simulink library "sm_vehicle_utilities_lib"  (R2024b)
settings: Solver=VariableStepAuto  StartTime=0.0  StopTime=10.0  RelTol=1e-3
undefined symbols (not defined in the file): Camera, Init, LorR, mu_surface, p1, p2, Scene_Data, SceneData, tire_data_205_60R19, vehdata, X, Y, Z
libraries: sm_lib x90, nesl_utility x49, $bdroot x33, fl_lib x10, simulink x8
(part 2 of 3)

== system sm_vehicle_utilities_lib/Mesh ==
  Solid : sm_lib/Body Elements/Extruded Solid  ExtrusionType=General  PolygonNumSides=3  PolygonOuterRadius=1  PolygonOuterRadiusUnits=m  ExportEntireGeometry=off  ExtrusionCrossSection=mesh_xsec  ExtrusionCrossSectionUnits=m  ExportConvexHullGeometry=off  ExtrusionLength=mesh_thickness  ExtrusionLengthUnits=m  InertiaType=CalculateFromGeometry  BasedOnType=Density  Density=mesh_rho  DensityUnits=kg/(m^3)  Mass=1  MassUnits=kg  CenterOfMass=[0 0 0]  CenterOfMassUnits=m  MomentsOfInertia=[1 1 1]  MomentsOfInertiaUnits=kg*m^2  ProductsOfInertia=[0 0 0]  ProductsOfInertiaUnits=kg*m^2  GraphicType=FromGeometry  MarkerShape=Sphere  MarkerSize=10  GraphicVisPropType=SimpleVisualProperties  GraphicDiffuseColor=mesh_color  GraphicOpacity=mesh_opc  GraphicSpecularColor=[0.5 0.5 0.5 1.0]  GraphicAmbientColor=[0.15 0.15 0.15 1.0]  GraphicEmissiveColor=[0.0 0.0 0.0 1.0]  GraphicShininess=75  DoExposeReferenceFrame=on  SerializedFrames=<Frames><Frame><Id>Frame1</Id><Value><Name>F</Name><Origin><Source>GeometricFeature</Source><FeatureName>top surface</FeatureName></Origin><PrimaryAxis><DefinedDirection>+Z</DefinedDirection><Source>ReferenceFrame</Source><SourceDirection>+Z</SourceDirection><FeatureName></FeatureName></PrimaryAxis><SecondaryAxis><DefinedDirection>+X</DefinedDirection><Source>ReferenceFrame</Source><SourceDirection>+X</SourceDirection><FeatureName></FeatureName></SecondaryAxis></Value></Frame><Frame><Id>Frame2</Id><Value><Name>B</Name><Origin><Source>GeometricFeature</Source><FeatureName>bottom surface</FeatureName></Origin><PrimaryAxis><DefinedDirection>+Z</DefinedDirection><Source>ReferenceFrame</Source><SourceDirection>+Z</SourceDirection><FeatureName></FeatureName></PrimaryAxis><SecondaryAxis><DefinedDirection>+X</DefinedDirection><Source>ReferenceFrame</Source><SourceDirection>+X</SourceDirection><FeatureName></FeatureName></SecondaryAxis></Value></Frame></Frames>
  F : PMIOPort  Side=Right
  R : PMIOPort  Port=2  Side=Left
  B : PMIOPort  Port=3  Side=Right
  connections:
  B/RConn1 -- Solid/LConn2
  F/RConn1 -- Solid/LConn1
  Solid/RConn1 -- R/RConn1

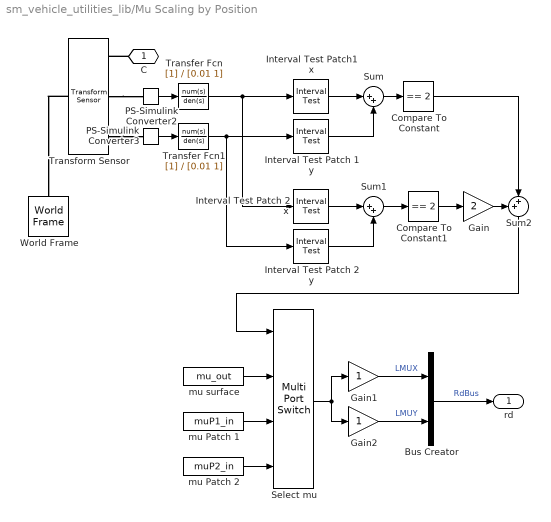
== system sm_vehicle_utilities_lib/Mu Scaling by Position ==
  Bus Creator : BusCreator  Inputs=2
  Compare To Constant : simulink/Logic and Bit Operations/Compare To Constant  relop===  const=2  OutDataTypeStr=boolean  ZeroCross=off
  Compare To Constant1 : simulink/Logic and Bit Operations/Compare To Constant  relop===  const=2  OutDataTypeStr=boolean  ZeroCross=off
  Gain : Gain  Gain=2
  Gain1 : Gain
  Gain2 : Gain
  Interval Test Patch 1 y : simulink/Logic and Bit Operations/Interval Test  IntervalClosedRight=on  uplimit=intvY_P1_end  IntervalClosedLeft=on  lowlimit=intvY_P1_start  OutDataTypeStr=uint8
  Interval Test Patch 2 x : simulink/Logic and Bit Operations/Interval Test  IntervalClosedRight=on  uplimit=intvX_P2_end  IntervalClosedLeft=on  lowlimit=intvX_P2_start  OutDataTypeStr=uint8
  Interval Test Patch 2 y : simulink/Logic and Bit Operations/Interval Test  IntervalClosedRight=on  uplimit=intvY_P2_end  IntervalClosedLeft=on  lowlimit=intvY_P2_start  OutDataTypeStr=uint8
  Interval Test Patch1 x : simulink/Logic and Bit Operations/Interval Test  IntervalClosedRight=on  uplimit=intvX_P1_end  IntervalClosedLeft=on  lowlimit=intvX_P1_start  OutDataTypeStr=uint8
  PS-Simulink Converter2 : nesl_utility/PS-Simulink Converter  PhysicalDomain=network_engine_domain  SubClassName=ps_output  LeftPortType=input  RightPortType=output  PseudoPeriodic=off  Frequencies=[]  VectorFormat=inherit  Unit=inherit  AffineConversion=off
  PS-Simulink Converter3 : nesl_utility/PS-Simulink Converter  PhysicalDomain=network_engine_domain  SubClassName=ps_output  LeftPortType=input  RightPortType=output  PseudoPeriodic=off  Frequencies=[]  VectorFormat=inherit  Unit=inherit  AffineConversion=off
  Select mu : MultiPortSwitch  DataPortOrder=Zero-based contiguous  zeroidx=on  SaturateOnIntegerOverflow=off  InputSameDT=off
  Sum : Sum  Inputs=|++
  Sum1 : Sum  Inputs=|++
  Sum2 : Sum  Inputs=++|
  Transfer Fcn : TransferFcn  Denominator=[0.01 1]
  Transfer Fcn1 : TransferFcn  Denominator=[0.01 1]
  Transform Sensor : sm_lib/Frames and Transforms/Transform Sensor  MeasurementFrame=World  RotationSequence=XYX  SenseAngle=off  SenseAxis=off  SenseQ=off  SenseR=off  SenseRotationSequence=off  SenseOmegaX=off  SenseOmegaY=off  SenseOmegaZ=off  SenseOmega=off  SenseQDot=off  SenseRDot=off  SenseRotationSequenceDot=off  SenseAlphaX=off  SenseAlphaY=off  SenseAlphaZ=off  SenseAlpha=off  SenseQDDot=off  SenseRDDot=off  SenseX=on  SenseY=on  SenseZ=off  SenseXYZ=off  SenseRad=off  SenseAzim=off  SenseDist=off  SenseInc=off  SenseXDot=off  SenseYDot=off  SenseZDot=off  SenseXYZDot=off  SenseRadDot=off  SenseAzimDot=off  SenseDistDot=off  SenseIncDot=off  SenseXDDot=off  SenseYDDot=off  SenseZDDot=off  SenseXYZDDot=off  SenseRadDDot=off  SenseAzimDDot=off  SenseDistDDot=off  SenseIncDDot=off
  World Frame : sm_lib/Frames and Transforms/World Frame
  mu Patch 1 : Constant  Value=muP1_in
  mu Patch 2 : Constant  Value=muP2_in
  mu surface : Constant  Value=mu_out
  C : PMIOPort  Side=Right
  rd : Outport  VectorParamsAs1DForOutWhenUnconnected=off
  wires:
  Interval Test Patch 2 y/1 -> Sum1/2
  Transfer Fcn1/1 -> Interval Test Patch 2 y/1, Interval Test Patch 1 y/1
  Sum1/1 -> Compare To Constant1/1
  Transfer Fcn/1 -> Interval Test Patch 2 x/1, Interval Test Patch1 x/1
  Interval Test Patch 2 x/1 -> Sum1/1
  Interval Test Patch1 x/1 -> Sum/1
  Interval Test Patch 1 y/1 -> Sum/2
  Sum/1 -> Compare To Constant/1
  Compare To Constant1/1 -> Gain/1
  mu surface/1 -> Select mu/2
  mu Patch 1/1 -> Select mu/3
  mu Patch 2/1 -> Select mu/4
  Sum2/1 -> Select mu/1
  Select mu/1 -> Gain2/1, Gain1/1
  Gain1/1 -> Bus Creator/1  "LMUX"
  Gain2/1 -> Bus Creator/2  "LMUY"
  Bus Creator/1 -> rd/1  "RdBus"
  Compare To Constant/1 -> Sum2/2
  Gain/1 -> Sum2/1
  PS-Simulink Converter2/1 -> Transfer Fcn/1
  PS-Simulink Converter3/1 -> Transfer Fcn1/1
  connections:
  C/RConn1 -- Transform Sensor/RConn1
  Transform Sensor/LConn1 -- World Frame/RConn1
  Transform Sensor/RConn2 -- PS-Simulink Converter2/LConn1
  Transform Sensor/RConn3 -- PS-Simulink Converter3/LConn1

== system sm_vehicle_utilities_lib/Pad Rotor ==
  note: Separate hard stop blocks are used so that we can measure only the pressure the piston applies to the rotor and so that we can have different stiffness values for piston-rotor and piston-caliper housing.
  note: Newtons
  note: Pascal
  Force Sensor : fl_lib/Mechanical/Mechanical Sensors/Ideal Force Sensor
  Hard Stop Caliper : fl_lib/Mechanical/Translational Elements/Translational Hard Stop  upper_bnd=0.1 m  lower_bnd=0 m  model=1  stiff_up=1e6 N/m  stiff_low=1e6 N/m  D_up=150 N/(m/s)  D_low=150 N/(m/s)  transition=0.1 mm  coeff_rest=0.7  v_tol=0.001 m/s  f_tol=0.001 N  v_specify=off  v_priority=None  v=0 m/s  v_nominal_specify=off  v_nominal_value=1  v_nominal_unit=m/s  f_specify=off  f_priority=None  f=0 N  f_nominal_specify=off  f_nominal_value=1  f_nominal_unit=N  x_specify=off  x_priority=High  x=0 m  x_nominal_specify=off  x_nominal_value=1  x_nominal_unit=m  M_specify=off  M_priority=None  M=0
  Hard Stop Rotor : fl_lib/Mechanical/Translational Elements/Translational Hard Stop  upper_bnd=0.45*1e-3 m  lower_bnd=-0.1 m  model=1  stiff_up=1e9*1e-3 N/m  stiff_low=1e9*1e-3 N/m  D_up=1e6*1e-3 N/(m/s)  D_low=1e6*1e-3 N/(m/s)  transition=0.045*1e-3 m  coeff_rest=0.7  v_tol=0.001 m/s  f_tol=0.001 N  v_specify=off  v_priority=None  v=0 m/s  v_nominal_specify=off  v_nominal_value=1  v_nominal_unit=m/s  f_specify=off  f_priority=None  f=0 N  f_nominal_specify=off  f_nominal_value=1  f_nominal_unit=N  x_specify=off  x_priority=High  x=0 m  x_nominal_specify=off  x_nominal_value=1  x_nominal_unit=m  M_specify=off  M_priority=None  M=0
  MTRef : fl_lib/Mechanical/Translational Elements/Mechanical Translational Reference
  MTRef1 : fl_lib/Mechanical/Translational Elements/Mechanical Translational Reference
  Mass : fl_lib/Mechanical/Translational Elements/Mass  mass=0.3 kg  num_ports=foundation.enum.numPorts2.one  v_specify=off  v_priority=High  v=0 m/s  v_nominal_specify=off  v_nominal_value=1  v_nominal_unit=m/s  f_specify=off  f_priority=None  f=0 N  f_nominal_specify=off  f_nominal_value=1  f_nominal_unit=N
  PS Calc Pressure Rotor : fl_lib/Physical Signals/Functions/PS Divide
  PS Cyl A : Subsystem
  pPad : PMIOPort  Side=Left
  Piston : PMIOPort  Port=2  Side=Right
  connections:
  PS Calc Pressure Rotor/RConn1 -- pPad/RConn1
  PS Calc Pressure Rotor/LConn2 -- PS Cyl A/RConn1
  PS Calc Pressure Rotor/LConn1 -- Force Sensor/RConn2
  Hard Stop Rotor/RConn1 -- Force Sensor/LConn1
  Force Sensor/RConn1 -- MTRef/LConn1
  Piston/RConn1 -- Hard Stop Rotor/LConn1 -- Hard Stop Caliper/LConn1 -- Mass/LConn1
  MTRef1/LConn1 -- Hard Stop Caliper/RConn1

== system sm_vehicle_utilities_lib/Plateau ==
  PS-Simulink Converter2 : nesl_utility/PS-Simulink Converter  PhysicalDomain=network_engine_domain  SubClassName=ps_output  LeftPortType=input  RightPortType=output  PseudoPeriodic=off  Frequencies=[]  VectorFormat=inherit  Unit=inherit  AffineConversion=off
  PS-Simulink Converter3 : nesl_utility/PS-Simulink Converter  PhysicalDomain=network_engine_domain  SubClassName=ps_output  LeftPortType=input  RightPortType=output  PseudoPeriodic=off  Frequencies=[]  VectorFormat=inherit  Unit=inherit  AffineConversion=off
  Road : Subsystem
  Transfer Fcn : TransferFcn  Denominator=[0.01 1]
  Transfer Fcn1 : TransferFcn  Denominator=[0.01 1]
  Transform Sensor : sm_lib/Frames and Transforms/Transform Sensor  MeasurementFrame=World  RotationSequence=XYX  SenseAngle=off  SenseAxis=off  SenseQ=off  SenseR=off  SenseRotationSequence=off  SenseOmegaX=off  SenseOmegaY=off  SenseOmegaZ=off  SenseOmega=off  SenseQDot=off  SenseRDot=off  SenseRotationSequenceDot=off  SenseAlphaX=off  SenseAlphaY=off  SenseAlphaZ=off  SenseAlpha=off  SenseQDDot=off  SenseRDDot=off  SenseX=on  SenseY=on  SenseZ=off  SenseXYZ=off  SenseRad=off  SenseAzim=off  SenseDist=off  SenseInc=off  SenseXDot=off  SenseYDot=off  SenseZDot=off  SenseXYZDot=off  SenseRadDot=off  SenseAzimDot=off  SenseDistDot=off  SenseIncDot=off  SenseXDDot=off  SenseYDDot=off  SenseZDDot=off  SenseXYZDDot=off  SenseRadDDot=off  SenseAzimDDot=off  SenseDistDDot=off  SenseIncDDot=off
  World Frame : sm_lib/Frames and Transforms/World Frame
  C : PMIOPort  Side=Right
  rd : Outport
  wires:
  PS-Simulink Converter2/1 -> Transfer Fcn/1
  PS-Simulink Converter3/1 -> Transfer Fcn1/1
  Road/1(R) -> rd/1
  Transfer Fcn/1 -> Road/1(x)
  Transfer Fcn1/1 -> Road/2(y)
  connections:
  Transform Sensor/LConn1 -- World Frame/RConn1
  Transform Sensor/RConn2 -- PS-Simulink Converter2/LConn1
  C/RConn1 -- Transform Sensor/RConn1
  Transform Sensor/RConn3 -- PS-Simulink Converter3/LConn1

== system sm_vehicle_utilities_lib/Position Camera Frame ==
  Transform Camera Frame : sm_lib/Frames and Transforms/Rigid Transform  RotationMethod=RotationSequence  FollAlignAxisA=+X  BaseAlignAxisA=+Y  FollAlignAxisB=+Y  BaseAlignAxisB=+Z  RotationStandardAxis=+Z  RotationAngle=0.0  RotationAngleUnits=deg  RotationArbitraryAxis=[0 0 1]  RotationSequenceAxes=FollowerAxes  RotationSequence=ZYX  RotationSequenceAngles=CF.a.Value(3:-1:1)  RotationSequenceAnglesUnits=deg  RotationMatrix=[1 0 0; 0 1 0; 0 0 1]  Quaternion=[1 0 0 0]  TranslationMethod=Cartesian  TranslationCartesianOffset=CF.s.Value  TranslationCartesianOffsetUnits=m  TranslationStandardAxis=+Z  TranslationStandardOffset=0  TranslationStandardOffsetUnits=m  TranslationROffset=0  TranslationROffsetUnits=m  TranslationThetaOffset=0  TranslationThetaOffsetUnits=deg  TranslationZOffset=0  TranslationZOffsetUnits=m
  B : PMIOPort  Side=Left
  F : PMIOPort  Port=2  Side=Right
  connections:
  Transform Camera Frame/LConn1 -- B/RConn1
  Transform Camera Frame/RConn1 -- F/RConn1

== system sm_vehicle_utilities_lib/Road ==
  note: This implementation is for a flat road
  Bus Creator1 : BusCreator  Inputs=8
  Constant : Constant  Value=SceneData.Reference.roll
  Constant{1,3,5..7} (5 alike) : Constant  Value=0
  Constant2 : Constant  Value=SceneData.Reference.yaw
  Constant4 : Constant  Value=SceneData.Reference.pitch
  R : Outport
  wires:
  Constant1/1 -> Bus Creator1/1  "px"
  Constant3/1 -> Bus Creator1/3  "pz"
  Constant5/1 -> Bus Creator1/2  "py"
  Constant/1 -> Bus Creator1/4  "qx"
  Constant2/1 -> Bus Creator1/6  "qz"
  Bus Creator1/1 -> R/1
  Constant4/1 -> Bus Creator1/5  "qy"
  Constant6/1 -> Bus Creator1/7  "LMUX"
  Constant7/1 -> Bus Creator1/8  "LMUY"

== system sm_vehicle_utilities_lib/Road Surface ==
  Flat : $bdroot/Flat  SystemSampleTime=-1  VariantControl=Flat  VariantActivationTime=update diagram  AllowFlexibleInterface=on  Latency=0  AutoFrameSizeCalculation=off
  Plateau : $bdroot/Plateau  VariantControl=Plateau  LRind=LorR
  Rough Road : $bdroot/Rough Road  VariantControl=Rough_Road  LRind=LorR
  C : PMIOPort  Side=Right
  rd : Outport

== system sm_vehicle_utilities_lib/Rough Road ==
  PS-Simulink Converter2 : nesl_utility/PS-Simulink Converter  PhysicalDomain=network_engine_domain  SubClassName=ps_output  LeftPortType=input  RightPortType=output  PseudoPeriodic=off  Frequencies=[]  VectorFormat=inherit  Unit=inherit  AffineConversion=off
  PS-Simulink Converter3 : nesl_utility/PS-Simulink Converter  PhysicalDomain=network_engine_domain  SubClassName=ps_output  LeftPortType=input  RightPortType=output  PseudoPeriodic=off  Frequencies=[]  VectorFormat=inherit  Unit=inherit  AffineConversion=off
  Road : Subsystem
  Transfer Fcn : TransferFcn  Denominator=[0.01 1]
  Transfer Fcn1 : TransferFcn  Denominator=[0.01 1]
  Transform Sensor : sm_lib/Frames and Transforms/Transform Sensor  MeasurementFrame=World  RotationSequence=XYX  SenseAngle=off  SenseAxis=off  SenseQ=off  SenseR=off  SenseRotationSequence=off  SenseOmegaX=off  SenseOmegaY=off  SenseOmegaZ=off  SenseOmega=off  SenseQDot=off  SenseRDot=off  SenseRotationSequenceDot=off  SenseAlphaX=off  SenseAlphaY=off  SenseAlphaZ=off  SenseAlpha=off  SenseQDDot=off  SenseRDDot=off  SenseX=on  SenseY=on  SenseZ=off  SenseXYZ=off  SenseRad=off  SenseAzim=off  SenseDist=off  SenseInc=off  SenseXDot=off  SenseYDot=off  SenseZDot=off  SenseXYZDot=off  SenseRadDot=off  SenseAzimDot=off  SenseDistDot=off  SenseIncDot=off  SenseXDDot=off  SenseYDDot=off  SenseZDDot=off  SenseXYZDDot=off  SenseRadDDot=off  SenseAzimDDot=off  SenseDistDDot=off  SenseIncDDot=off
  World Frame : sm_lib/Frames and Transforms/World Frame
  C : PMIOPort  Side=Right
  rd : Outport
  wires:
  Transfer Fcn1/1 -> Road/2(y)
  Transfer Fcn/1 -> Road/1(x)
  Road/1(R) -> rd/1
  PS-Simulink Converter3/1 -> Transfer Fcn1/1
  PS-Simulink Converter2/1 -> Transfer Fcn/1
  connections:
  Transform Sensor/RConn3 -- PS-Simulink Converter3/LConn1
  C/RConn1 -- Transform Sensor/RConn1
  Transform Sensor/RConn2 -- PS-Simulink Converter2/LConn1
  Transform Sensor/LConn1 -- World Frame/RConn1

== system sm_vehicle_utilities_lib/Scene Plateau ==
  RDF Polyline : Subsystem  mask{road_extr_data_L=RDF_Polyline.Road.extr_data_L, road_extr_data_R=RDF_Polyline.Road.extr_data_R, road_profile_sep=RDF_Polyline.Road.profile_separation, road_w=RDF_Polyline.Road.w, road_x=RDF_Polyline.Road.x, road_z=RDF_Polyline.Road.z, road_yaw=RDF_Polyline.Road.yaw, road_clr=RDF_Polyline.Road.clr, road_opc=RDF_Polyline.Road.opc}
      mask prompts: road_extr_data_L "Road Profile Left [x y] (m)"; road_extr_data_R "Road Profile Right [x y] (m)"; road_profile_sep "Profile Separation (m)"; road_w "Width (m)"; road_x "Offset x (m)"; road_z "Offset z (m)"; road_yaw "Offset yaw (rad)"; road_clr "Color [R G B]"; road_opc "Opacity (0-1)"
  W : PMIOPort  Side=Left
  connections:
  W/RConn1 -- RDF Polyline/RConn1

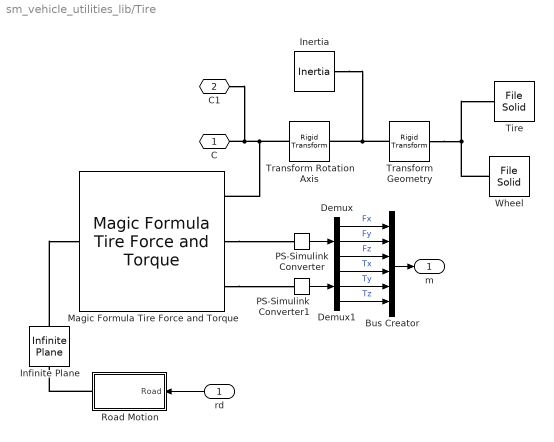
== system sm_vehicle_utilities_lib/Tire ==
  rd : Inport
  Bus Creator : BusCreator  Inputs=6
  Demux : Demux  Outputs=3
  Demux1 : Demux  Outputs=3
  Inertia : sm_lib/Body Elements/Inertia  InertiaType=Custom  Mass=wheelbody_mass  MassUnits=kg  CenterOfMass=[0 0 0]  CenterOfMassUnits=m  MomentsOfInertia=wheelbody_I  MomentsOfInertiaUnits=kg*m^2  ProductsOfInertia=[0 0 0]  ProductsOfInertiaUnits=kg*m^2  GraphicType=None  MarkerShape=Inertia  MarkerSize=20  GraphicVisPropType=SimpleVisualProperties  GraphicDiffuseColor=[0.5 0.5 0.5]  GraphicOpacity=1.0  GraphicSpecularColor=[0.5 0.5 0.5 1.0]  GraphicAmbientColor=[0.15 0.15 0.15 1.0]  GraphicEmissiveColor=[0.0 0.0 0.0 1.0]  GraphicShininess=75
  Infinite Plane : sm_lib/Curves and Surfaces/Infinite Plane  GraphicType=Rectangle  GraphicPlaneWidth=1  GraphicPlaneWidthUnits=m  GraphicPlaneHeight=1  GraphicPlaneHeightUnits=m  GraphicVisPropType=SimpleVisualProperties  GraphicDiffuseColor=[0.5 0.5 0.5]  GraphicOpacity=0.25  GraphicSpecularColor=[0.5 0.5 0.5 1.0]  GraphicAmbientColor=[0.15 0.15 0.15 1.0]  GraphicEmissiveColor=[0.0 0.0 0.0 1.0]  GraphicShininess=75
  Magic Formula Tire Force and Torque : sm_lib/Forces and Torques/Magic Formula Tire Force and Torque  TireSide=Left  TireParameters=tire_param  SlipMode=Combined  ContactFrameMethod=ClosestPoint  ScalingCoefficientLMUXMode=FromTireParameters  ScalingCoefficientLMUYMode=FromTireParameters  SenseContactSignal=off  TireWrenchFrame=ContactFrame  SenseTireForce=on  SenseTireTorque=on  SensePneumaticTrail=off  SenseLongitudinalSlip=off  SenseSaturatedLongitudinalSlip=off  SenseSlipAngle=off  SenseSaturatedSlipAngle=off  SenseTurnSlip=off  SenseRelativeLongitudinalVelocity=off  SenseRelativeLateralVelocity=off  SenseLongitudinalSlipVelocity=off  SenseLateralSlipVelocity=off  SenseYawVelocity=off  SenseCamberAngle=off  SenseSaturatedCamberAngle=off  SenseCamberVelocity=off  SenseSpinVelocity=off  SenseFreeRadius=off  SenseLoadedRadius=off  SenseEffectiveRollingRadius=off  SenseRadialDeflection=off  SenseLongitudinalFrictionCoefficient=off  SenseLateralFrictionCoefficient=off  SenseContactBaseRotation=off  SenseContactBaseTranslation=off  SenseContactFollowerRotation=off  SenseContactFollowerTranslation=off  NumericParameters=[0.1 0.1 0.1 0.1 5.0 1e-4 1e-4 1e-7 1e-7 1e-4 1e-4 0.1 1e-4 1e-4 1e-4 1e-4 1e-4 1e-4 1e-4 1e-4 1e-4]
  PS-Simulink Converter : nesl_utility/PS-Simulink Converter  PhysicalDomain=network_engine_domain  SubClassName=ps_output  LeftPortType=input  RightPortType=output  PseudoPeriodic=off  Frequencies=[]  VectorFormat=1-D array  Unit=inherit  AffineConversion=off
  PS-Simulink Converter1 : nesl_utility/PS-Simulink Converter  PhysicalDomain=network_engine_domain  SubClassName=ps_output  LeftPortType=input  RightPortType=output  PseudoPeriodic=off  Frequencies=[]  VectorFormat=1-D array  Unit=inherit  AffineConversion=off
  Road Motion : Subsystem
  Tire : sm_lib/Body Elements/File Solid  ExtGeomFileName=sm_vehicle_slalom_tire.STL  UnitType=Custom  ExtGeomFileUnits=mm  StepReaderType=HEX  ExportConvexHullGeometry=off  InertiaType=Custom  BasedOnType=Density  Density=1000  DensityUnits=kg/m^3  Mass=0  MassUnits=kg  CenterOfMass=[0 0 0]  CenterOfMassUnits=m  MomentsOfInertia=[0 0 0]  MomentsOfInertiaUnits=kg*m^2  ProductsOfInertia=[0 0 0]  ProductsOfInertiaUnits=kg*m^2  GraphicType=FromGeometry  MarkerShape=Sphere  MarkerSize=10  GraphicVisPropType=SimpleVisualProperties  GraphicDiffuseColor=[0.5 0.5 0.5]  GraphicOpacity=1.0  GraphicSpecularColor=[0.5 0.5 0.5 1.0]  GraphicAmbientColor=[0.15 0.15 0.15 1.0]  GraphicEmissiveColor=[0.0 0.0 0.0 1.0]  GraphicShininess=75  DoExposeReferenceFrame=on  SerializedFrames=<Frames/>
  Transform Geometry : sm_lib/Frames and Transforms/Rigid Transform  RotationMethod=StandardAxis  FollAlignAxisA=+X  BaseAlignAxisA=+Y  FollAlignAxisB=+Y  BaseAlignAxisB=+Z  RotationStandardAxis=+X  RotationAngle=180*side_lr-90  RotationAngleUnits=deg  RotationArbitraryAxis=[0 0 1]  RotationSequenceAxes=FollowerAxes  RotationSequence=XYX  RotationSequenceAngles=[0 0 0]  RotationSequenceAnglesUnits=deg  RotationMatrix=[1 0 0; 0 1 0; 0 0 1]  Quaternion=[1 0 0 0]  TranslationMethod=StandardAxis  TranslationCartesianOffset=[0 0 0]  TranslationCartesianOffsetUnits=m  TranslationStandardAxis=+Y  TranslationStandardOffset=(1-2*side_lr)*0.125  TranslationStandardOffsetUnits=m  TranslationROffset=0  TranslationROffsetUnits=m  TranslationThetaOffset=0  TranslationThetaOffsetUnits=deg  TranslationZOffset=0  TranslationZOffsetUnits=m
  Transform Rotation Axis : sm_lib/Frames and Transforms/Rigid Transform  RotationMethod=AlignedAxes  FollAlignAxisA=+X  BaseAlignAxisA=+X  FollAlignAxisB=+Z  BaseAlignAxisB=+Y  RotationStandardAxis=+Z  RotationAngle=0.0  RotationAngleUnits=deg  RotationArbitraryAxis=[0 0 1]  RotationSequenceAxes=FollowerAxes  RotationSequence=XYX  RotationSequenceAngles=[0 0 0]  RotationSequenceAnglesUnits=deg  RotationMatrix=[1 0 0; 0 1 0; 0 0 1]  Quaternion=[1 0 0 0]  TranslationMethod=None  TranslationCartesianOffset=[0 0 0]  TranslationCartesianOffsetUnits=m  TranslationStandardAxis=+Z  TranslationStandardOffset=0  TranslationStandardOffsetUnits=m  TranslationROffset=0  TranslationROffsetUnits=m  TranslationThetaOffset=0  TranslationThetaOffsetUnits=deg  TranslationZOffset=0  TranslationZOffsetUnits=m
  Wheel : sm_lib/Body Elements/File Solid  ExtGeomFileName=sm_vehicle_slalom_wheel.STL  UnitType=Custom  ExtGeomFileUnits=mm  StepReaderType=HEX  ExportConvexHullGeometry=off  InertiaType=Custom  BasedOnType=Density  Density=1000  DensityUnits=kg/m^3  Mass=0  MassUnits=kg  CenterOfMass=[0 0 0]  CenterOfMassUnits=m  MomentsOfInertia=[0 0 0]  MomentsOfInertiaUnits=kg*m^2  ProductsOfInertia=[0 0 0]  ProductsOfInertiaUnits=kg*m^2  GraphicType=FromGeometry  MarkerShape=Sphere  MarkerSize=10  GraphicVisPropType=SimpleVisualProperties  GraphicDiffuseColor=[0.8 0.8 0.8]  GraphicOpacity=1.0  GraphicSpecularColor=[0.5 0.5 0.5 1.0]  GraphicAmbientColor=[0.15 0.15 0.15 1.0]  GraphicEmissiveColor=[0.0 0.0 0.0 1.0]  GraphicShininess=75  DoExposeReferenceFrame=on  SerializedFrames=<Frames/>
  C : PMIOPort  Side=Left
  C1 : PMIOPort  Port=2  Side=Left
  m : Outport
  wires:
  PS-Simulink Converter/1 -> Demux/1
  Demux/1 -> Bus Creator/1  "Fx"
  Demux/2 -> Bus Creator/2  "Fy"
  Demux/3 -> Bus Creator/3  "Fz"
  Demux1/3 -> Bus Creator/6  "Tz"
  Demux1/2 -> Bus Creator/5  "Ty"
  Demux1/1 -> Bus Creator/4  "Tx"
  PS-Simulink Converter1/1 -> Demux1/1
  Bus Creator/1 -> m/1
  rd/1 -> Road Motion/1(Road)
  connections:
  Wheel/RConn1 -- Transform Geometry/RConn1 -- Tire/RConn1
  C1/RConn1 -- Magic Formula Tire Force and Torque/RConn1 -- Transform Rotation Axis/RConn1 -- C/RConn1
  Infinite Plane/RConn1 -- Magic Formula Tire Force and Torque/LConn1
  Magic Formula Tire Force and Torque/RConn2 -- PS-Simulink Converter/LConn1
  Magic Formula Tire Force and Torque/RConn3 -- PS-Simulink Converter1/LConn1
  Road Motion/RConn1 -- Infinite Plane/LConn1
  Inertia/RConn1 -- Transform Rotation Axis/LConn1 -- Transform Geometry/LConn1

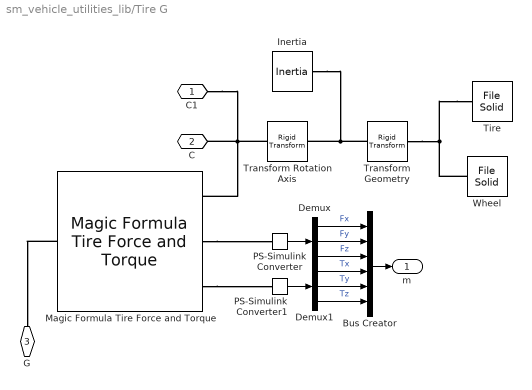
== system sm_vehicle_utilities_lib/Tire G ==
  Bus Creator : BusCreator  Inputs=6
  Demux : Demux  Outputs=3
  Demux1 : Demux  Outputs=3
  Inertia : sm_lib/Body Elements/Inertia  InertiaType=Custom  Mass=wheelbody_mass  MassUnits=kg  CenterOfMass=[0 0 0]  CenterOfMassUnits=m  MomentsOfInertia=wheelbody_I  MomentsOfInertiaUnits=kg*m^2  ProductsOfInertia=[0 0 0]  ProductsOfInertiaUnits=kg*m^2  GraphicType=None  MarkerShape=Inertia  MarkerSize=20  GraphicVisPropType=SimpleVisualProperties  GraphicDiffuseColor=[0.5 0.5 0.5]  GraphicOpacity=1.0  GraphicSpecularColor=[0.5 0.5 0.5 1.0]  GraphicAmbientColor=[0.15 0.15 0.15 1.0]  GraphicEmissiveColor=[0.0 0.0 0.0 1.0]  GraphicShininess=75
  Magic Formula Tire Force and Torque : sm_lib/Forces and Torques/Magic Formula Tire Force and Torque  TireSide=Left  TireParameters=tire_param  SlipMode=Combined  ContactFrameMethod=ClosestPoint  ScalingCoefficientLMUXMode=FromTireParameters  ScalingCoefficientLMUYMode=FromTireParameters  SenseContactSignal=off  TireWrenchFrame=ContactFrame  SenseTireForce=on  SenseTireTorque=on  SensePneumaticTrail=off  SenseLongitudinalSlip=off  SenseSaturatedLongitudinalSlip=off  SenseSlipAngle=off  SenseSaturatedSlipAngle=off  SenseTurnSlip=off  SenseRelativeLongitudinalVelocity=off  SenseRelativeLateralVelocity=off  SenseLongitudinalSlipVelocity=off  SenseLateralSlipVelocity=off  SenseYawVelocity=off  SenseCamberAngle=off  SenseSaturatedCamberAngle=off  SenseCamberVelocity=off  SenseSpinVelocity=off  SenseFreeRadius=off  SenseLoadedRadius=off  SenseEffectiveRollingRadius=off  SenseRadialDeflection=off  SenseLongitudinalFrictionCoefficient=off  SenseLateralFrictionCoefficient=off  SenseContactBaseRotation=off  SenseContactBaseTranslation=off  SenseContactFollowerRotation=off  SenseContactFollowerTranslation=off  NumericParameters=[0.1 0.1 0.1 0.1 5.0 1e-4 1e-4 1e-7 1e-7 1e-4 1e-4 0.1 1e-4 1e-4 1e-4 1e-4 1e-4 1e-4 1e-4 1e-4 1e-4]
  PS-Simulink Converter : nesl_utility/PS-Simulink Converter  PhysicalDomain=network_engine_domain  SubClassName=ps_output  LeftPortType=input  RightPortType=output  PseudoPeriodic=off  Frequencies=[]  VectorFormat=1-D array  Unit=inherit  AffineConversion=off
  PS-Simulink Converter1 : nesl_utility/PS-Simulink Converter  PhysicalDomain=network_engine_domain  SubClassName=ps_output  LeftPortType=input  RightPortType=output  PseudoPeriodic=off  Frequencies=[]  VectorFormat=1-D array  Unit=inherit  AffineConversion=off
  Tire : sm_lib/Body Elements/File Solid  ExtGeomFileName=sm_vehicle_slalom_tire.STL  UnitType=Custom  ExtGeomFileUnits=mm  StepReaderType=HEX  ExportConvexHullGeometry=off  InertiaType=Custom  BasedOnType=Density  Density=1000  DensityUnits=kg/m^3  Mass=0  MassUnits=kg  CenterOfMass=[0 0 0]  CenterOfMassUnits=m  MomentsOfInertia=[0 0 0]  MomentsOfInertiaUnits=kg*m^2  ProductsOfInertia=[0 0 0]  ProductsOfInertiaUnits=kg*m^2  GraphicType=FromGeometry  MarkerShape=Sphere  MarkerSize=10  GraphicVisPropType=SimpleVisualProperties  GraphicDiffuseColor=[0.5 0.5 0.5]  GraphicOpacity=1.0  GraphicSpecularColor=[0.5 0.5 0.5 1.0]  GraphicAmbientColor=[0.15 0.15 0.15 1.0]  GraphicEmissiveColor=[0.0 0.0 0.0 1.0]  GraphicShininess=75  DoExposeReferenceFrame=on  SerializedFrames=<Frames/>
  Transform Geometry : sm_lib/Frames and Transforms/Rigid Transform  RotationMethod=StandardAxis  FollAlignAxisA=+X  BaseAlignAxisA=+Y  FollAlignAxisB=+Y  BaseAlignAxisB=+Z  RotationStandardAxis=+X  RotationAngle=180*side_lr-90  RotationAngleUnits=deg  RotationArbitraryAxis=[0 0 1]  RotationSequenceAxes=FollowerAxes  RotationSequence=XYX  RotationSequenceAngles=[0 0 0]  RotationSequenceAnglesUnits=deg  RotationMatrix=[1 0 0; 0 1 0; 0 0 1]  Quaternion=[1 0 0 0]  TranslationMethod=StandardAxis  TranslationCartesianOffset=[0 0 0]  TranslationCartesianOffsetUnits=m  TranslationStandardAxis=+Y  TranslationStandardOffset=(1-2*side_lr)*0.125  TranslationStandardOffsetUnits=m  TranslationROffset=0  TranslationROffsetUnits=m  TranslationThetaOffset=0  TranslationThetaOffsetUnits=deg  TranslationZOffset=0  TranslationZOffsetUnits=m
  Transform Rotation Axis : sm_lib/Frames and Transforms/Rigid Transform  RotationMethod=AlignedAxes  FollAlignAxisA=+X  BaseAlignAxisA=+X  FollAlignAxisB=+Z  BaseAlignAxisB=+Y  RotationStandardAxis=+Z  RotationAngle=0.0  RotationAngleUnits=deg  RotationArbitraryAxis=[0 0 1]  RotationSequenceAxes=FollowerAxes  RotationSequence=XYX  RotationSequenceAngles=[0 0 0]  RotationSequenceAnglesUnits=deg  RotationMatrix=[1 0 0; 0 1 0; 0 0 1]  Quaternion=[1 0 0 0]  TranslationMethod=None  TranslationCartesianOffset=[0 0 0]  TranslationCartesianOffsetUnits=m  TranslationStandardAxis=+Z  TranslationStandardOffset=0  TranslationStandardOffsetUnits=m  TranslationROffset=0  TranslationROffsetUnits=m  TranslationThetaOffset=0  TranslationThetaOffsetUnits=deg  TranslationZOffset=0  TranslationZOffsetUnits=m
  Wheel : sm_lib/Body Elements/File Solid  ExtGeomFileName=sm_vehicle_slalom_wheel.STL  UnitType=Custom  ExtGeomFileUnits=mm  StepReaderType=HEX  ExportConvexHullGeometry=off  InertiaType=Custom  BasedOnType=Density  Density=1000  DensityUnits=kg/m^3  Mass=0  MassUnits=kg  CenterOfMass=[0 0 0]  CenterOfMassUnits=m  MomentsOfInertia=[0 0 0]  MomentsOfInertiaUnits=kg*m^2  ProductsOfInertia=[0 0 0]  ProductsOfInertiaUnits=kg*m^2  GraphicType=FromGeometry  MarkerShape=Sphere  MarkerSize=10  GraphicVisPropType=SimpleVisualProperties  GraphicDiffuseColor=[0.8 0.8 0.8]  GraphicOpacity=1.0  GraphicSpecularColor=[0.5 0.5 0.5 1.0]  GraphicAmbientColor=[0.15 0.15 0.15 1.0]  GraphicEmissiveColor=[0.0 0.0 0.0 1.0]  GraphicShininess=75  DoExposeReferenceFrame=on  SerializedFrames=<Frames/>
  C1 : PMIOPort  Side=Left
  C : PMIOPort  Port=2  Side=Left
  G : PMIOPort  Port=3  Side=Left
  m : Outport
  wires:
  Bus Creator/1 -> m/1
  PS-Simulink Converter1/1 -> Demux1/1
  Demux1/1 -> Bus Creator/4  "Tx"
  Demux1/2 -> Bus Creator/5  "Ty"
  Demux1/3 -> Bus Creator/6  "Tz"
  Demux/3 -> Bus Creator/3  "Fz"
  Demux/2 -> Bus Creator/2  "Fy"
  Demux/1 -> Bus Creator/1  "Fx"
  PS-Simulink Converter/1 -> Demux/1
  connections:
  Transform Geometry/LConn1 -- Transform Rotation Axis/LConn1 -- Inertia/RConn1
  Magic Formula Tire Force and Torque/RConn3 -- PS-Simulink Converter1/LConn1
  Magic Formula Tire Force and Torque/RConn2 -- PS-Simulink Converter/LConn1
  Magic Formula Tire Force and Torque/LConn1 -- G/RConn1
  C/RConn1 -- C1/RConn1 -- Transform Rotation Axis/RConn1 -- Magic Formula Tire Force and Torque/RConn1
  Tire/RConn1 -- Transform Geometry/RConn1 -- Wheel/RConn1

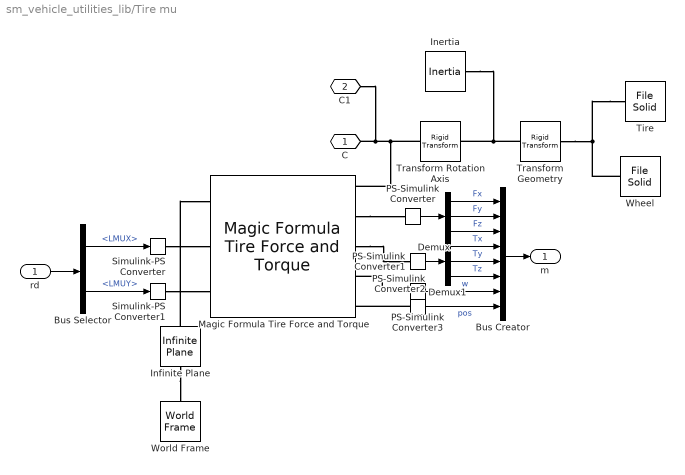
== system sm_vehicle_utilities_lib/Tire mu ==
  rd : Inport
  Bus Creator : BusCreator  Inputs=8
  Bus Selector : BusSelector  OutputSignals=LMUX,LMUY
  Demux : Demux  Outputs=3
  Demux1 : Demux  Outputs=3
  Inertia : sm_lib/Body Elements/Inertia  InertiaType=Custom  Mass=wheelbody_mass  MassUnits=kg  CenterOfMass=[0 0 0]  CenterOfMassUnits=m  MomentsOfInertia=wheelbody_I  MomentsOfInertiaUnits=kg*m^2  ProductsOfInertia=[0 0 0]  ProductsOfInertiaUnits=kg*m^2  GraphicType=None  MarkerShape=Inertia  MarkerSize=20  GraphicVisPropType=SimpleVisualProperties  GraphicDiffuseColor=[0.5 0.5 0.5]  GraphicOpacity=1.0  GraphicSpecularColor=[0.5 0.5 0.5 1.0]  GraphicAmbientColor=[0.15 0.15 0.15 1.0]  GraphicEmissiveColor=[0.0 0.0 0.0 1.0]  GraphicShininess=75
  Infinite Plane : sm_lib/Curves and Surfaces/Infinite Plane  GraphicType=Rectangle  GraphicPlaneWidth=1  GraphicPlaneWidthUnits=m  GraphicPlaneHeight=1  GraphicPlaneHeightUnits=m  GraphicVisPropType=SimpleVisualProperties  GraphicDiffuseColor=[0.5 0.5 0.5]  GraphicOpacity=0.25  GraphicSpecularColor=[0.5 0.5 0.5 1.0]  GraphicAmbientColor=[0.15 0.15 0.15 1.0]  GraphicEmissiveColor=[0.0 0.0 0.0 1.0]  GraphicShininess=75
  Magic Formula Tire Force and Torque : sm_lib/Forces and Torques/Magic Formula Tire Force and Torque  TireSide=Left  TireParameters=tire_param  SlipMode=Combined  ContactFrameMethod=ClosestPoint  ScalingCoefficientLMUXMode=ProvidedByInput  ScalingCoefficientLMUYMode=ProvidedByInput  SenseContactSignal=off  TireWrenchFrame=ContactFrame  SenseTireForce=on  SenseTireTorque=on  SensePneumaticTrail=off  SenseLongitudinalSlip=off  SenseSaturatedLongitudinalSlip=off  SenseSlipAngle=off  SenseSaturatedSlipAngle=off  SenseTurnSlip=off  SenseRelativeLongitudinalVelocity=off  SenseRelativeLateralVelocity=off  SenseLongitudinalSlipVelocity=off  SenseLateralSlipVelocity=off  SenseYawVelocity=off  SenseCamberAngle=off  SenseSaturatedCamberAngle=off  SenseCamberVelocity=off  SenseSpinVelocity=on  SenseFreeRadius=off  SenseLoadedRadius=off  SenseEffectiveRollingRadius=off  SenseRadialDeflection=off  SenseLongitudinalFrictionCoefficient=off  SenseLateralFrictionCoefficient=off  SenseContactBaseRotation=off  SenseContactBaseTranslation=on  SenseContactFollowerRotation=off  SenseContactFollowerTranslation=off  NumericParameters=[0.1 0.1 0.1 0.1 5.0 1e-4 1e-4 1e-7 1e-7 1e-4 1e-4 0.1 1e-4 1e-4 1e-4 1e-4 1e-4 1e-4 1e-4 1e-4 1e-4]
  PS-Simulink Converter{,1..3} (4 alike) : nesl_utility/PS-Simulink Converter  PhysicalDomain=network_engine_domain  SubClassName=ps_output  LeftPortType=input  RightPortType=output  PseudoPeriodic=off  Frequencies=[]  VectorFormat=1-D array  Unit=inherit  AffineConversion=off
  Simulink-PS Converter : nesl_utility/Simulink-PS Converter  PhysicalDomain=network_engine_domain  SubClassName=ps_input  LeftPortType=input  RightPortType=output  PseudoPeriodic=off  Frequencies=[]  NoiseDistribution=none  NoiseParameters=[]  Unit=1  AffineConversion=off  FilteringAndDerivatives=provide  SimscapeFilterOrder=1  InputFilterTimeConstant=0.001  UdotUserProvided=0
  Simulink-PS Converter1 : nesl_utility/Simulink-PS Converter  PhysicalDomain=network_engine_domain  SubClassName=ps_input  LeftPortType=input  RightPortType=output  PseudoPeriodic=off  Frequencies=[]  NoiseDistribution=none  NoiseParameters=[]  Unit=1  AffineConversion=off  FilteringAndDerivatives=provide  SimscapeFilterOrder=1  InputFilterTimeConstant=0.001  UdotUserProvided=0
  Tire : sm_lib/Body Elements/File Solid  ExtGeomFileName=sm_vehicle_slalom_tire.STL  UnitType=Custom  ExtGeomFileUnits=mm  StepReaderType=HEX  ExportConvexHullGeometry=off  InertiaType=Custom  BasedOnType=Density  Density=1000  DensityUnits=kg/m^3  Mass=0  MassUnits=kg  CenterOfMass=[0 0 0]  CenterOfMassUnits=m  MomentsOfInertia=[0 0 0]  MomentsOfInertiaUnits=kg*m^2  ProductsOfInertia=[0 0 0]  ProductsOfInertiaUnits=kg*m^2  GraphicType=FromGeometry  MarkerShape=Sphere  MarkerSize=10  GraphicVisPropType=SimpleVisualProperties  GraphicDiffuseColor=[0.5 0.5 0.5]  GraphicOpacity=1.0  GraphicSpecularColor=[0.5 0.5 0.5 1.0]  GraphicAmbientColor=[0.15 0.15 0.15 1.0]  GraphicEmissiveColor=[0.0 0.0 0.0 1.0]  GraphicShininess=75  DoExposeReferenceFrame=on  SerializedFrames=<Frames/>
  Transform Geometry : sm_lib/Frames and Transforms/Rigid Transform  RotationMethod=StandardAxis  FollAlignAxisA=+X  BaseAlignAxisA=+Y  FollAlignAxisB=+Y  BaseAlignAxisB=+Z  RotationStandardAxis=+X  RotationAngle=180*side_lr-90  RotationAngleUnits=deg  RotationArbitraryAxis=[0 0 1]  RotationSequenceAxes=FollowerAxes  RotationSequence=XYX  RotationSequenceAngles=[0 0 0]  RotationSequenceAnglesUnits=deg  RotationMatrix=[1 0 0; 0 1 0; 0 0 1]  Quaternion=[1 0 0 0]  TranslationMethod=StandardAxis  TranslationCartesianOffset=[0 0 0]  TranslationCartesianOffsetUnits=m  TranslationStandardAxis=+Y  TranslationStandardOffset=(1-2*side_lr)*0.125  TranslationStandardOffsetUnits=m  TranslationROffset=0  TranslationROffsetUnits=m  TranslationThetaOffset=0  TranslationThetaOffsetUnits=deg  TranslationZOffset=0  TranslationZOffsetUnits=m
  Transform Rotation Axis : sm_lib/Frames and Transforms/Rigid Transform  RotationMethod=AlignedAxes  FollAlignAxisA=+X  BaseAlignAxisA=+X  FollAlignAxisB=+Z  BaseAlignAxisB=+Y  RotationStandardAxis=+Z  RotationAngle=0.0  RotationAngleUnits=deg  RotationArbitraryAxis=[0 0 1]  RotationSequenceAxes=FollowerAxes  RotationSequence=XYX  RotationSequenceAngles=[0 0 0]  RotationSequenceAnglesUnits=deg  RotationMatrix=[1 0 0; 0 1 0; 0 0 1]  Quaternion=[1 0 0 0]  TranslationMethod=None  TranslationCartesianOffset=[0 0 0]  TranslationCartesianOffsetUnits=m  TranslationStandardAxis=+Z  TranslationStandardOffset=0  TranslationStandardOffsetUnits=m  TranslationROffset=0  TranslationROffsetUnits=m  TranslationThetaOffset=0  TranslationThetaOffsetUnits=deg  TranslationZOffset=0  TranslationZOffsetUnits=m
  Wheel : sm_lib/Body Elements/File Solid  ExtGeomFileName=sm_vehicle_slalom_wheel.STL  UnitType=Custom  ExtGeomFileUnits=mm  StepReaderType=HEX  ExportConvexHullGeometry=off  InertiaType=Custom  BasedOnType=Density  Density=1000  DensityUnits=kg/m^3  Mass=0  MassUnits=kg  CenterOfMass=[0 0 0]  CenterOfMassUnits=m  MomentsOfInertia=[0 0 0]  MomentsOfInertiaUnits=kg*m^2  ProductsOfInertia=[0 0 0]  ProductsOfInertiaUnits=kg*m^2  GraphicType=FromGeometry  MarkerShape=Sphere  MarkerSize=10  GraphicVisPropType=SimpleVisualProperties  GraphicDiffuseColor=[0.8 0.8 0.8]  GraphicOpacity=1.0  GraphicSpecularColor=[0.5 0.5 0.5 1.0]  GraphicAmbientColor=[0.15 0.15 0.15 1.0]  GraphicEmissiveColor=[0.0 0.0 0.0 1.0]  GraphicShininess=75  DoExposeReferenceFrame=on  SerializedFrames=<Frames/>
  World Frame : sm_lib/Frames and Transforms/World Frame
  C : PMIOPort  Side=Left
  C1 : PMIOPort  Port=2  Side=Left
  m : Outport
  wires:
  rd/1 -> Bus Selector/1
  Bus Creator/1 -> m/1
  PS-Simulink Converter1/1 -> Demux1/1
  Demux1/1 -> Bus Creator/4  "Tx"
  Demux1/2 -> Bus Creator/5  "Ty"
  Demux1/3 -> Bus Creator/6  "Tz"
  Demux/3 -> Bus Creator/3  "Fz"
  Demux/2 -> Bus Creator/2  "Fy"
  Demux/1 -> Bus Creator/1  "Fx"
  PS-Simulink Converter/1 -> Demux/1
  Bus Selector/1 -> Simulink-PS Converter/1  "<LMUX>"
  Bus Selector/2 -> Simulink-PS Converter1/1  "<LMUY>"
  PS-Simulink Converter2/1 -> Bus Creator/8  "pos"
  PS-Simulink Converter3/1 -> Bus Creator/7  "w"
  connections:
  Transform Geometry/LConn1 -- Transform Rotation Axis/LConn1 -- Inertia/RConn1
  Infinite Plane/LConn1 -- World Frame/RConn1
  Magic Formula Tire Force and Torque/RConn3 -- PS-Simulink Converter1/LConn1
  Magic Formula Tire Force and Torque/RConn2 -- PS-Simulink Converter/LConn1
  Infinite Plane/RConn1 -- Magic Formula Tire Force and Torque/LConn1
  C/RConn1 -- Transform Rotation Axis/RConn1 -- Magic Formula Tire Force and Torque/RConn1 -- C1/RConn1
  Tire/RConn1 -- Transform Geometry/RConn1 -- Wheel/RConn1
  Simulink-PS Converter/RConn1 -- Magic Formula Tire Force and Torque/LConn2
  Simulink-PS Converter1/RConn1 -- Magic Formula Tire Force and Torque/LConn3
  PS-Simulink Converter2/LConn1 -- Magic Formula Tire Force and Torque/RConn5
  PS-Simulink Converter3/LConn1 -- Magic Formula Tire Force and Torque/RConn4

== system sm_vehicle_utilities_lib/Valve Control ==
  Slip : Inport
  vSpdEst : Inport  Port=2
  Categorize Surface : Subsystem
  Code to Valves : Subsystem
  Demux : Demux  Outputs=2
  Logic : Stateflow chart  TreatAsAtomicUnit=on
  Mux : Mux  Inputs=2
  Product : Product
  Subsystem : Subsystem
  Subsystem1 : Subsystem
  Valve : Outport  VectorParamsAs1DForOutWhenUnconnected=off
  wires:
  Logic/1(Mod_State) -> Categorize Surface/1(Mod State), Code to Valves/1(C)
  Logic/2(Mod_Dur) -> Product/2
  Slip/1 -> Logic/1(Slip)
  Code to Valves/1(V) -> Product/1
  vSpdEst/1 -> Logic/2(vSpdEst)
  Product/1 -> Demux/1
  Demux/1 -> Subsystem/1(OnT)
  Demux/2 -> Subsystem1/1(OnT)
  Mux/1 -> Valve/1
  Subsystem/1(vSig) -> Mux/1, Categorize Surface/2(Apply Valve)
  Subsystem1/1(vSig) -> Mux/2

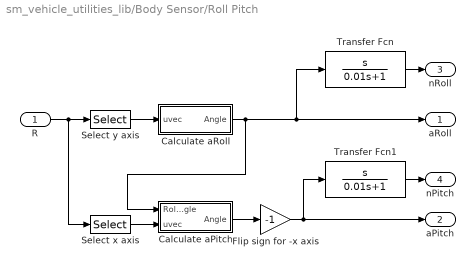
== system sm_vehicle_utilities_lib/Body Sensor/Roll Pitch ==
  R : Inport
  Calculate aPitch : Subsystem
  Calculate aRoll : Subsystem
  "Flip sign for -x axis " : Gain  Gain=-1
  Select x axis : Selector  NumberOfDimensions=2  InputPortWidth=2  IndexOptions=Index vector (dialog),Index vector (dialog)  Indices=[1 2 3],1  OutputSizes=1,1
  Select y axis : Selector  NumberOfDimensions=2  InputPortWidth=2  IndexOptions=Index vector (dialog),Index vector (dialog)  Indices=[1 2 3],2  OutputSizes=1,1
  Transfer Fcn : TransferFcn  Numerator=[1 0]  Denominator=[0.01 1]
  Transfer Fcn1 : TransferFcn  Numerator=[1 0]  Denominator=[0.01 1]
  aRoll : Outport  VectorParamsAs1DForOutWhenUnconnected=off
  aPitch : Outport  Port=2  VectorParamsAs1DForOutWhenUnconnected=off
  nRoll : Outport  Port=3  VectorParamsAs1DForOutWhenUnconnected=off
  nPitch : Outport  Port=4  VectorParamsAs1DForOutWhenUnconnected=off
  wires:
  Transfer Fcn1/1 -> nPitch/1
  Transfer Fcn/1 -> nRoll/1
  Calculate aRoll/1(Angle) -> Calculate aPitch/1(Roll Angle), aRoll/1, Transfer Fcn/1
  "Flip sign for -x axis "/1 -> Transfer Fcn1/1, aPitch/1
  Select y axis/1 -> Calculate aRoll/1(uvec)
  R/1 -> Select x axis/1, Select y axis/1
  Select x axis/1 -> Calculate aPitch/2(uvec)
  Calculate aPitch/1(Angle) -> "Flip sign for -x axis "/1

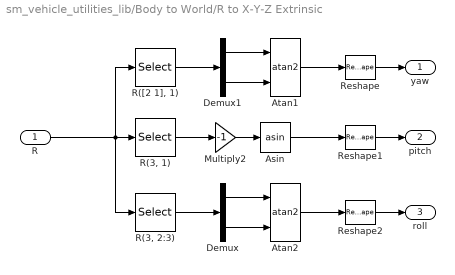
== system sm_vehicle_utilities_lib/Body to World/R to X-Y-Z Extrinsic ==
  R : Inport
  Asin : Trigonometry  Operator=asin
  Atan1 : Trigonometry  Operator=atan2
  Atan2 : Trigonometry  Operator=atan2
  Demux : Demux  Outputs=2
  Demux1 : Demux  Outputs=2
  Multiply2 : Gain  Gain=-1
  "R(3, 1)" : Selector  NumberOfDimensions=2  InputPortWidth=3  IndexOptions=Index vector (dialog),Index vector (dialog)  Indices=3,1  OutputSizes=1,1
  "R(3, 2:3)" : Selector  NumberOfDimensions=2  InputPortWidth=3  IndexOptions=Index vector (dialog),Index vector (dialog)  Indices=3,[2 3]  OutputSizes=1,1
  "R([2 1], 1)" : Selector  NumberOfDimensions=2  InputPortWidth=3  IndexOptions=Index vector (dialog),Index vector (dialog)  Indices=[2 1],1  OutputSizes=1,1
  Reshape : Reshape
  Reshape1 : Reshape
  Reshape2 : Reshape  OutputDimensionality=Customize  OutputDimensions=1
  yaw : Outport  VectorParamsAs1DForOutWhenUnconnected=off
  pitch : Outport  Port=2  VectorParamsAs1DForOutWhenUnconnected=off
  roll : Outport  Port=3  VectorParamsAs1DForOutWhenUnconnected=off
  wires:
  Demux/1 -> Atan2/1
  Demux1/2 -> Atan1/2
  Demux/2 -> Atan2/2
  Atan2/1 -> Reshape2/1
  "R(3, 1)"/1 -> Multiply2/1
  Asin/1 -> Reshape1/1
  R/1 -> "R(3, 1)"/1, "R(3, 2:3)"/1, "R([2 1], 1)"/1
  Demux1/1 -> Atan1/1
  "R([2 1], 1)"/1 -> Demux1/1
  Multiply2/1 -> Asin/1
  "R(3, 2:3)"/1 -> Demux/1
  Atan1/1 -> Reshape/1
  Reshape/1 -> yaw/1
  Reshape1/1 -> pitch/1
  Reshape2/1 -> roll/1

== system sm_vehicle_utilities_lib/Camera Frames/Dolly Camera ==
  Off : Subsystem  VariantControl=Off  mask{tvec=Camera.Dolly_Cam.tvec.Value, xvec=Camera.Dolly_Cam.xvec.Value, yvec=Camera.Dolly_Cam.yvec.Value, zvec=Camera.Dolly_Cam.zvec.Value, s=Camera.Dolly_Cam.s.Value, a=Camera.Dolly_Cam.a.Value}
      mask prompts: tvec "Time Vector (s)"; xvec "X Vector (m)"; yvec "Y Vector (m)"; zvec "Z Vector (m)"; s "Camera Offset [xyz] (m)"; a "Camera Orientation [Roll-Pitch-Yaw] (deg)"
  XYZ : Subsystem  VariantControl=XYZ  mask{tvec=Camera.Dolly_Cam.tvec.Value, xvec=Camera.Dolly_Cam.xvec.Value, yvec=Camera.Dolly_Cam.yvec.Value, zvec=Camera.Dolly_Cam.zvec.Value, s=Camera.Dolly_Cam.s.Value, a=Camera.Dolly_Cam.a.Value}
      mask prompts: tvec "Time Vector (s)"; xvec "X Vector (m)"; yvec "Y Vector (m)"; zvec "Z Vector (m)"; s "Camera Offset [xyz] (m)"; a "Camera Orientation [Roll-Pitch-Yaw] (deg)"
  " W" : PMIOPort  Side=Left
  " R" : PMIOPort  Port=2  Side=Right

== system sm_vehicle_utilities_lib/Flat/Road ==
  note: This implementation is for a flat road
  Bus Creator1 : BusCreator  Inputs=8
  Constant : Constant  Value=SceneData.Reference.roll
  Constant1 : Constant  Value=0
  Constant2 : Constant  Value=SceneData.Reference.yaw
  Constant3 : Constant  Value=0
  Constant4 : Constant  Value=SceneData.Reference.pitch
  Constant5 : Constant  Value=0
  Constant6 : Constant
  Constant7 : Constant
  R : Outport
  wires:
  Constant4/1 -> Bus Creator1/5  "qy"
  Bus Creator1/1 -> R/1
  Constant2/1 -> Bus Creator1/6  "qz"
  Constant/1 -> Bus Creator1/4  "qx"
  Constant5/1 -> Bus Creator1/2  "py"
  Constant3/1 -> Bus Creator1/3  "pz"
  Constant1/1 -> Bus Creator1/1  "px"
  Constant7/1 -> Bus Creator1/7  "LMUX"
  Constant6/1 -> Bus Creator1/8  "LMUY"

== system sm_vehicle_utilities_lib/Pad Rotor/PS Cyl A ==
  PS Constant : fl_lib/Physical Signals/Sources/PS Constant  constant=d_caliper_piston m
  PS Gain pi div 4 : fl_lib/Physical Signals/Functions/PS Gain  gain=pi/4
  PS Product1 : fl_lib/Physical Signals/Functions/PS Product
  cylA : PMIOPort  Side=Right
  connections:
  PS Gain pi div 4/RConn1 -- cylA/RConn1
  PS Gain pi div 4/LConn1 -- PS Product1/RConn1
  PS Constant/RConn1 -- PS Product1/LConn1 -- PS Product1/LConn2

== system sm_vehicle_utilities_lib/Plateau/Road ==
  note: This implementation only varies road height and pitch along World x-axis.
  x : Inport
  y : Inport  Port=2
  1-D Lookup Table pitch : Lookup_n-D  NumberOfTableDimensions=1  BreakpointsForDimension1=SceneData.Plateau.Road.qyLUT.px  Table=SceneData.Plateau.Road.qyLUT.qy(:,LRind)  InterpMethod=Akima spline  InternalRulePriority=Speed  RndMeth=Simplest
  1-D Lookup Table pz : Lookup_n-D  NumberOfTableDimensions=1  BreakpointsForDimension1=SceneData.Plateau.Road.pzLUT.px  Table=SceneData.Plateau.Road.pzLUT.pz(:,LRind)  InterpMethod=Akima spline  InternalRulePriority=Speed  RndMeth=Simplest
  Bus Creator1 : BusCreator  Inputs=6
  Constant : Constant  Value=0
  Constant2 : Constant  Value=0
  R : Outport
  wires:
  x/1 -> Bus Creator1/1, 1-D Lookup Table pz/1, 1-D Lookup Table pitch/1  "px"
  y/1 -> Bus Creator1/2  "py"
  Constant/1 -> Bus Creator1/4  "qx"
  Constant2/1 -> Bus Creator1/6  "qz"
  Bus Creator1/1 -> R/1
  1-D Lookup Table pitch/1 -> Bus Creator1/5  "qy"
  1-D Lookup Table pz/1 -> Bus Creator1/3  "pz"

== system sm_vehicle_utilities_lib/Rough Road/Road ==
  note: This implementation only varies road height and pitch along World x-axis.
  x : Inport
  y : Inport  Port=2
  1-D Lookup Table pitch : Lookup_n-D  NumberOfTableDimensions=1  BreakpointsForDimension1=SceneData.Rough_Road.Road.qyLUT.px  Table=SceneData.Rough_Road.Road.qyLUT.qy(:,LRind)  InterpMethod=Akima spline  InternalRulePriority=Speed  RndMeth=Simplest
  1-D Lookup Table pz : Lookup_n-D  NumberOfTableDimensions=1  BreakpointsForDimension1=SceneData.Rough_Road.Road.pzLUT.px  Table=SceneData.Rough_Road.Road.pzLUT.pz(:,LRind)  InterpMethod=Akima spline  InternalRulePriority=Speed  RndMeth=Simplest
  Bus Creator1 : BusCreator  Inputs=6
  Constant : Constant  Value=0
  Constant2 : Constant  Value=0
  R : Outport
  wires:
  1-D Lookup Table pz/1 -> Bus Creator1/3  "pz"
  1-D Lookup Table pitch/1 -> Bus Creator1/5  "qy"
  Bus Creator1/1 -> R/1
  Constant2/1 -> Bus Creator1/6  "qz"
  Constant/1 -> Bus Creator1/4  "qx"
  y/1 -> Bus Creator1/2  "py"
  x/1 -> 1-D Lookup Table pitch/1, 1-D Lookup Table pz/1, Bus Creator1/1  "px"
